simulink model "sfcndemo_timestwo"  (Simulink 7.6)
settings: Solver=FixedStepDiscrete  StartTime=0.0  StopTime=10.0  RelTol=1e-3
Description:
  | Simple C-Mex S-function
settings Model: Creator=The MathWorks Inc.  ExtModeTrigMode=oneshot  ExtModeArmWhenConnect=off  ExtModeAutoUpdateStatusClock=off
settings DataIOCC: LimitDataPoints=off
settings OptimizationCC: BlockReduction=off  BooleanDataType=off  InitFltsAndDblsToZero=on
settings DebuggingCC: SaveWithParameterizedLinksMsg=none  SignalResolutionControl=TryResolveAllWithWarning  SolverPrmCheckMsg=none  MultiTaskDSMMsg=warning  MultiTaskCondExecSysMsg=none
settings HardwareCC: TargetUnknown=on
settings RTWCC: IncludeERTFirstTime=on
settings CodeAppCC: CustomSymbolStrFcn=$F$N$M
settings GRTTargetCC: TargetFcnLib=ansi_tfl_tmw.mat

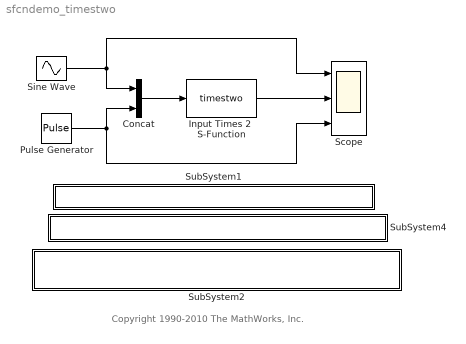
== system sfcndemo_timestwo ==
  note: Copyright 1990-2010 The MathWorks, Inc.
  Concat : Concatenate  Mode=Vector
  Input Times 2  S-Function : S-Function  FunctionName=timestwo  EnableBusSupport=off
  Pulse Generator : DiscretePulseGenerator  PulseType=Time based  Amplitude=1:3  Period=1  PulseWidth=50
  Scope : Scope  NumInputPorts=3
      settings: TimeRange=10  YMin=-2~-5~0  YMax=2~10~3
  Sine Wave : Sin  Amplitude=1:2  SampleTime=0
  SubSystem1 : Subsystem  mask{filename=timestwo.c}
      mask init:
      | x=sfundemo_maskdisp;
      settings: AttributesFormatString=\n  OpenFcn=sfundemo_openfcn
      mask Display: disp(x);
  SubSystem2 : Subsystem  mask{filename=timestwo.m}
      mask init:
      | x=sfundemo_maskdisp;
      settings: AttributesFormatString=\n  OpenFcn=sfundemo_openfcn
      mask Display: disp(['MATLAB file: ' x '\nNote:to run this file, please disable the executable mex file in your path.']);
  SubSystem4 : Subsystem  mask{filename=timestwo.tlc}
      mask init:
      | x=sfundemo_maskdisp;
      settings: AttributesFormatString=\n  OpenFcn=sfundemo_openfcn
      mask Display: disp(x);
  wires:
  Input Times 2  S-Function/1 -> Scope/2
  Concat/1 -> Input Times 2  S-Function/1
  Pulse Generator/1 -> Concat/2, Scope/3
  Sine Wave/1 -> Concat/1, Scope/1

== system sfcndemo_timestwo/SubSystem1 ==

== system sfcndemo_timestwo/SubSystem2 ==

== system sfcndemo_timestwo/SubSystem4 ==
